simulink model "teensyshot_test_1"  (R2018b)
settings: Solver=FixedStepDiscrete  StartTime=0.0  StopTime=Inf  RelTol=1e-3
libraries: rpi_blkst x1
settings Model: SimulationMode=external  Creator=jacques  LastModifiedBy=jacques
settings OptimizationCC: EnhancedBackFolding=on  PassReuseOutputArgsAs=Individual arguments  OptimizeBlockOrder=speed  DifferentSizesBufferReuse=on  OptimizationCustomize=off
settings DebuggingCC: ParameterTunabilityLossMsg=error
settings HardwareCC: ProdBitPerPointer=32  ProdBitPerSizeT=32  ProdBitPerPtrDiffT=32  ProdLargestAtomicInteger=Long  ProdLargestAtomicFloat=Double  ProdWordSize=32  ProdHWDeviceType=ARM Compatible->ARM 11
settings SFSimCC: MATLABDynamicMemAlloc=off
settings RTWCC: SystemTargetFile=ert_rpi.tlc  TemplateMakefile=ert_rpi.tmf  PostCodeGenCommand=postGenFunc(buildInfo)  Description=RTW Embedded Coder RPI target  GenerateReport=on  IncludeHyperlinkInReport=on  LaunchReport=on  GenerateTraceInfo=on  GenerateTraceReport=on  GenerateTraceReportSl=on  GenerateTraceReportSf=on  GenerateTraceReportEml=on
settings CodeAppCC: ForceParamTrailComments=on  IgnoreCustomStorageClasses=off  OperatorAnnotations=on  SimulinkDataObjDesc=on  SFDataObjDesc=on  InsertBlockDesc=on
settings STFCustomTargetCC: TargetLangStandard=C99 (ISO)  MultiwordLength=256  ModelReferenceCompliant=off  CombineOutputUpdateFcns=on  ERTCustomFileBanners=on  SupportNonInlinedSFcns=off  RemoveResetFunc=on  MATLABClassNameForMDSCustomization=Simulink.SoftwareTarget.ERTCustomization  SystemTargetFile=ert_rpi.tlc
settings ERTTargetCC: TargetLangStandard=C99 (ISO)  ModelReferenceCompliant=off  ParMdlRefBuildCompliant=off  CompOptLevelCompliant=off  ConcurrentExecutionCompliant=off  SupportContinuousTime=on  ModelStepFunctionPrototypeControlCompliant=off  CPPClassGenCompliant=off  UseToolchainInfoCompliant=off  ExtMode=on  ExtModeMexArgs='10.0.1.60'  ERTCustomFileTemplate=ert_rpi_file_process.tlc

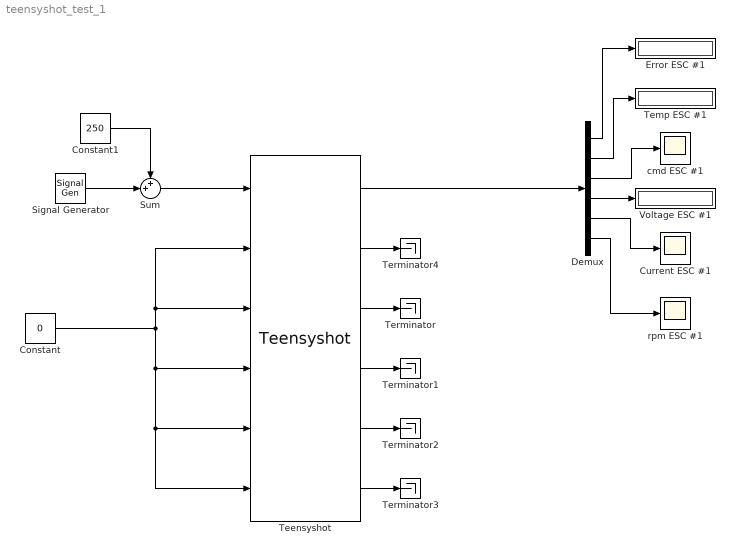
== system teensyshot_test_1 ==
  Constant : Constant  Value=0  SampleTime=0.01
  Constant1 : Constant  Value=250  SampleTime=0.01
  Current ESC #1 : Scope
  Demux : Demux  Outputs=6
  Error ESC #1 : Display
  Signal Generator : SignalGenerator  WaveForm=square  Amplitude=50  Frequency=0.25
  Sum : Sum  Inputs=++|
  Teensyshot : rpi_blkst/Teensyshot  rpi_mask_port=5488750  rpi_mask_Ts=0.01  rpi_mask_P1=1400.0  rpi_mask_I1=1600.0  rpi_mask_D1=4000.0  rpi_mask_f1=9900.0  rpi_mask_P2=400  rpi_mask_I2=1050  rpi_mask_D2=1000  rpi_mask_f2=9900  rpi_mask_P3=0  rpi_mask_I3=0  rpi_mask_D3=0  rpi_mask_f3=0  rpi_mask_P4=0  rpi_mask_I4=0  rpi_mask_D4=0  rpi_mask_f4=0  rpi_mask_P5=0  rpi_mask_I5=0  rpi_mask_D5=0  rpi_mask_f5=0  rpi_mask_P6=0  rpi_mask_I6=0  rpi_mask_D6=0  rpi_mask_f6=0
      settings: SourceProductName=RPI Blockset
  Temp ESC #1 : Display
  Terminator{,1..4} (5 alike) : Terminator
  Voltage ESC #1 : Display
  cmd ESC #1 : Scope
  rpm ESC #1 : Scope
  wires:
  Constant/1 -> Teensyshot/4, Teensyshot/5, Teensyshot/6, Teensyshot/3, Teensyshot/2
  Teensyshot/3 -> Terminator/1
  Teensyshot/4 -> Terminator1/1
  Teensyshot/5 -> Terminator2/1
  Teensyshot/6 -> Terminator3/1
  Teensyshot/1 -> Demux/1
  Demux/2 -> Temp ESC #1/1
  Demux/1 -> Error ESC #1/1
  Demux/3 -> cmd ESC #1/1
  Demux/4 -> Voltage ESC #1/1
  Demux/5 -> Current ESC #1/1
  Demux/6 -> rpm ESC #1/1
  Teensyshot/2 -> Terminator4/1
  Signal Generator/1 -> Sum/2
  Sum/1 -> Teensyshot/1
  Constant1/1 -> Sum/1
